simulink model "diagrama_de_bloques_actitud"  (R2017b)
settings: Solver=FixedStepDiscrete  StartTime=0.0  StopTime=erle.T_simulacion  FixedStep=erle.Tm  RelTol=1e-3
undefined symbols (not defined in the file or in its folder): erle
settings Model: Creator=javi  LastModifiedBy=javi
settings DataIOCC: SaveFormat=Array

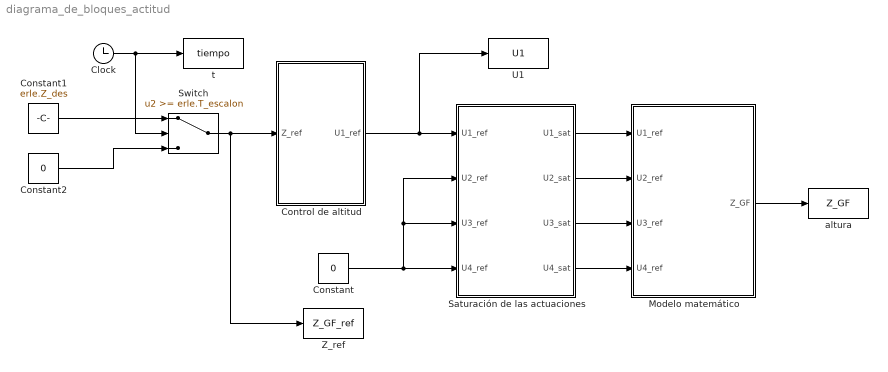
== system diagrama_de_bloques_actitud ==
  Clock : Clock
  Constant : Constant  Value=0
  Constant1 : Constant  Value=erle.Z_des
  Constant2 : Constant  Value=0
  Control de altitud : Subsystem
  Modelo matemático : Subsystem
  Saturación de las actuaciones : Subsystem
  Switch : Switch  Threshold=erle.T_escalon
  U1 : ToWorkspace  VariableName=U1  SampleTime=erle.Tm
  Z_ref : ToWorkspace  VariableName=Z_GF_ref  SampleTime=erle.Tm
  altura : ToWorkspace  VariableName=Z_GF  SampleTime=erle.Tm
  "t " : ToWorkspace  VariableName=tiempo  SampleTime=erle.Tm
  wires:
  Saturación de las actuaciones/1(U1_sat) -> Modelo matemático/1(U1_ref)
  Saturación de las actuaciones/2(U2_sat) -> Modelo matemático/2(U2_ref)
  Saturación de las actuaciones/3(U3_sat) -> Modelo matemático/3(U3_ref)
  Saturación de las actuaciones/4(U4_sat) -> Modelo matemático/4(U4_ref)
  Modelo matemático/1(Z_GF) -> altura/1
  Clock/1 -> Switch/2, "t "/1
  Constant/1 -> Saturación de las actuaciones/4(U4_ref), Saturación de las actuaciones/3(U3_ref), Saturación de las actuaciones/2(U2_ref)
  Switch/1 -> Z_ref/1, Control de altitud/1(Z_ref)
  Constant1/1 -> Switch/1
  Constant2/1 -> Switch/3
  Control de altitud/1(U1_ref) -> U1/1, Saturación de las actuaciones/1(U1_ref)

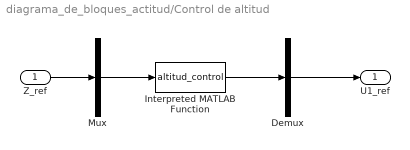
== system diagrama_de_bloques_actitud/Control de altitud ==
  Z_ref : Inport
  Demux : Demux  Outputs=1
  Interpreted MATLAB Function : MATLABFcn  MATLABFcn=altitud_control
  Mux : Mux  Inputs=1
  U1_ref : Outport
  wires:
  Interpreted MATLAB Function/1 -> Demux/1
  Demux/1 -> U1_ref/1
  Z_ref/1 -> Mux/1
  Mux/1 -> Interpreted MATLAB Function/1

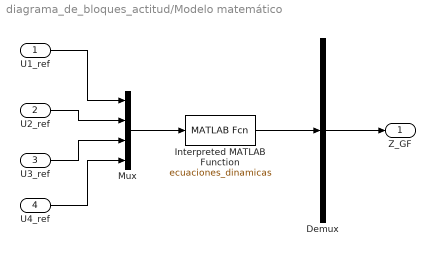
== system diagrama_de_bloques_actitud/Modelo matemático ==
  U1_ref : Inport
  U2_ref : Inport  Port=2
  U3_ref : Inport  Port=3
  U4_ref : Inport  Port=4
  Demux : Demux  Outputs=1
  Interpreted MATLAB Function : MATLABFcn  MATLABFcn=ecuaciones_dinamicas  OutputDimensions=1
  Mux : Mux
  Z_GF : Outport
  wires:
  U3_ref/1 -> Mux/3
  Mux/1 -> Interpreted MATLAB Function/1
  U2_ref/1 -> Mux/2
  U4_ref/1 -> Mux/4
  U1_ref/1 -> Mux/1
  Interpreted MATLAB Function/1 -> Demux/1
  Demux/1 -> Z_GF/1

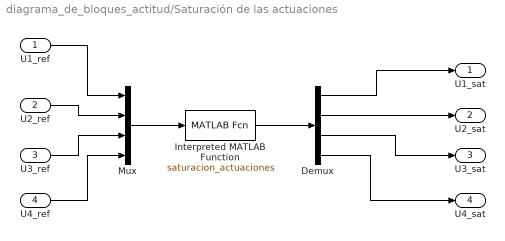
== system diagrama_de_bloques_actitud/Saturación de las actuaciones ==
  U1_ref : Inport
  U2_ref : Inport  Port=2
  U3_ref : Inport  Port=3
  U4_ref : Inport  Port=4
  Demux : Demux
  Interpreted MATLAB Function : MATLABFcn  MATLABFcn=saturacion_actuaciones  OutputDimensions=4
  Mux : Mux
  U1_sat : Outport
  U2_sat : Outport  Port=2
  U3_sat : Outport  Port=3
  U4_sat : Outport  Port=4
  wires:
  Demux/1 -> U1_sat/1
  Interpreted MATLAB Function/1 -> Demux/1
  Demux/2 -> U2_sat/1
  U3_ref/1 -> Mux/3
  Demux/3 -> U3_sat/1
  U4_ref/1 -> Mux/4
  U2_ref/1 -> Mux/2
  U1_ref/1 -> Mux/1
  Demux/4 -> U4_sat/1
  Mux/1 -> Interpreted MATLAB Function/1
